simulink model "mRobotArm_PickAndPlace"  (R2021a)
settings: Solver=FixedStepAuto  StartTime=0.0  StopTime=inf  RelTol=1e-3  EnableMultiTasking=on
InitFcn:
  | initPoint=[pi/2 pi/2 pi/4 pi/4];
  | placePoint = [2.3562 1.1920 0.4461 0.0025];
  | pickPoint = [130; -130; 10];
undefined symbols (not defined in the file or in its folder): adHome6deg, adHome6rad, adWS
libraries: arduinolib x13, aerolibconvert2 x2
settings Model: SILPILModeSetting=veronly  ExtModeTrigDuration=2  Creator=loris  LastModifiedBy=angelo
settings OptimizationCC: EnhancedBackFolding=on  PassReuseOutputArgsAs=Individual arguments  ZeroExternalMemoryAtStartup=off  ZeroInternalMemoryAtStartup=off  MaxStackSize=64  OptimizeBlockOrder=speed  DifferentSizesBufferReuse=on  OptimizationCustomize=off  EfficientTunableParamExpr=on
settings DebuggingCC: ParameterTunabilityLossMsg=error
settings HardwareCC: ProdBitPerInt=16  ProdBitPerPointer=16  ProdBitPerSizeT=16  ProdBitPerPtrDiffT=16  ProdLargestAtomicFloat=None  ProdWordSize=8  ProdHWDeviceType=Atmel->AVR
settings SFSimCC: MATLABDynamicMemAlloc=off
settings RTWCC: SystemTargetFile=ert.tlc  HardwareBoard=Arduino Mega 2560  TemplateMakefile=ert_default_tmf  Toolchain=Arduino AVR  BuildConfiguration=Faster Runs
settings CodeAppCC: ForceParamTrailComments=on  IgnoreCustomStorageClasses=off  OperatorAnnotations=on  SimulinkDataObjDesc=on  SFDataObjDesc=on  InsertBlockDesc=on
settings ERTTargetCC: SupportContinuousTime=on  SupportVariableSizeSignals=on  ExtModeStaticAllocSize=2048

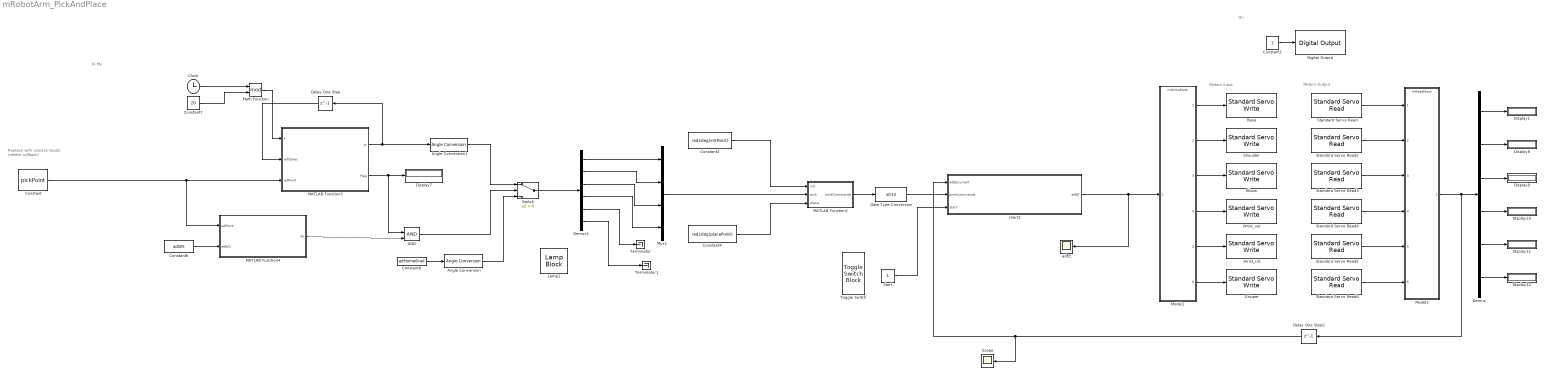
== system mRobotArm_PickAndPlace ==
  note: Replace with camera inputs
      | (delete callback)
  note: On
  note: Motors Output
  note: Motors Input
  note: IK My
  AND : Logic  IconShape=distinctive  AllPortsSameDT=off  OutDataTypeStr=boolean
  Angle Conversion : aerolibconvert2/Angle Conversion  IU=rad  OU=deg
  Angle Conversion1 : aerolibconvert2/Angle Conversion  IU=rad  OU=deg
  Base : arduinolib/Standard Servo Write  pinNumber=11  ServoIndex=0  blockPlatform=ARDUINO
  Clock : Clock
  Constant : Constant  Value=pickPoint
  Constant1 : Constant
  Constant3 : Constant  Value=rad2deg(initPoint)
  Constant4 : Constant  Value=rad2deg(placePoint)
  Constant6 : Constant  Value=adWS
  Constant7 : Constant  Value=20
  Constant8 : Constant  Value=adHome6rad
  Data Type Conversion : DataTypeConversion  OutDataTypeStr=int32
  Delay One Step : Delay  DelayLength=1  InitialCondition=adHome6rad  SampleTime=0.02
  Delay One Step2 : Delay  DelayLength=1  InitialCondition=adHome6deg
  Demux : Demux  Outputs=6
  Demux1 : Demux  Outputs=6
  Digital Output : arduinolib/Digital Output  pinNumber=12  Direction=output  blockPlatform=arduino
  Display{1,7..12} (7 alike) : Display
  Elbow : arduinolib/Standard Servo Write  pinNumber=9  ServoIndex=1  blockPlatform=ARDUINO
  Gripper : arduinolib/Standard Servo Write  pinNumber=3  ServoIndex=2  blockPlatform=ARDUINO
  Lamp1 : LampBlock  LabelPosition=Hide
  MATLAB Function1 : MATLAB Function  TreatAsAtomicUnit=on
  MATLAB Function3 : MATLAB Function  TreatAsAtomicUnit=on  SystemSampleTime=0.02
  MATLAB Function4 : MATLAB Function  TreatAsAtomicUnit=on  SystemSampleTime=0.02
  Math Function : Math  Operator=mod  SaturateOnIntegerOverflow=on
  Model1 : ModelReference  ModelNameDialog=mWriteMask.slx  SimulationMode=Normal  ModelReferenceVersion=1.1
  Model2 : ModelReference  ModelNameDialog=mReadMask.slx  SimulationMode=Normal  ModelReferenceVersion=1.1
  Mux1 : Mux
  Scope : Scope
  Shoulder : arduinolib/Standard Servo Write  pinNumber=10  ServoIndex=3  blockPlatform=ARDUINO
  Standard Servo Read : arduinolib/Standard Servo Read  pinNumber=11  SampleTime=0.02  ServoIndex=0  blockPlatform=ARDUINO
      settings: SourceProductBaseCode=ARDUINO
  Standard Servo Read2 : arduinolib/Standard Servo Read  pinNumber=10  SampleTime=0.02  ServoIndex=3  blockPlatform=ARDUINO
      settings: SourceProductBaseCode=ARDUINO
  Standard Servo Read3 : arduinolib/Standard Servo Read  pinNumber=9  SampleTime=0.02  ServoIndex=1  blockPlatform=ARDUINO
      settings: SourceProductBaseCode=ARDUINO
  Standard Servo Read4 : arduinolib/Standard Servo Read  pinNumber=6  SampleTime=0.02  ServoIndex=4  blockPlatform=ARDUINO
      settings: SourceProductBaseCode=ARDUINO
  Standard Servo Read5 : arduinolib/Standard Servo Read  pinNumber=5  SampleTime=0.02  ServoIndex=5  blockPlatform=ARDUINO
      settings: SourceProductBaseCode=ARDUINO
  Standard Servo Read6 : arduinolib/Standard Servo Read  pinNumber=3  SampleTime=0.02  ServoIndex=2  blockPlatform=ARDUINO
      settings: SourceProductBaseCode=ARDUINO
  Start : Constant
  Switch : Switch  Criteria=u2 > Threshold
  Terminator : Terminator
  Terminator1 : Terminator
  Toggle Switch : ToggleSwitchBlock  LabelPosition=Hide
      settings: Values={{'Off', 'On'}, [0 1]}
  Wrist_rot : arduinolib/Standard Servo Write  pinNumber=5  ServoIndex=5  blockPlatform=ARDUINO
  Wrist_ver : arduinolib/Standard Servo Write  pinNumber=6  ServoIndex=4  blockPlatform=ARDUINO
  adEE : Scope
  chart2 : Stateflow chart  TreatAsAtomicUnit=on  SystemSampleTime=0.02
  wires:
  Constant1/1 -> Digital Output/1
  Delay One Step2/1 -> Scope/1, chart2/1(adEEcurrent)
  Constant3/1 -> MATLAB Function1/1(init)
  Constant4/1 -> MATLAB Function1/3(place)
  MATLAB Function3/2(flag) -> Display7/1, AND/1
  Constant7/1 -> Math Function/2
  Constant6/1 -> MATLAB Function4/2(adWS)
  Clock/1 -> Math Function/1
  MATLAB Function3/1(jc) -> Delay One Step/1, Angle Conversion1/1
  Constant/1 -> MATLAB Function4/1(adPoint), MATLAB Function3/3(adPoint)
  Delay One Step/1 -> MATLAB Function3/2(adQprec)
  AND/1 -> Switch/2
  Math Function/1 -> MATLAB Function3/1(t)
  MATLAB Function4/1(ok) -> AND/2
  Demux1/1 -> Mux1/1
  Demux1/2 -> Mux1/2
  Demux1/3 -> Mux1/3
  Demux1/4 -> Mux1/4
  Mux1/1 -> MATLAB Function1/2(pick)
  Demux1/5 -> Terminator/1
  Switch/1 -> Demux1/1
  chart2/1(adEE) -> Model1/1, adEE/1
  Start/1 -> chart2/3(start)
  Demux/6 -> Display12/1
  Demux/2 -> Display8/1
  Demux/5 -> Display11/1
  Demux/4 -> Display10/1
  Demux/1 -> Display1/1
  Demux/3 -> Display9/1
  Model2/1 -> Delay One Step2/1, Demux/1
  Demux1/6 -> Terminator1/1
  MATLAB Function1/1(jointCommands) -> Data Type Conversion/1
  Data Type Conversion/1 -> chart2/2(JointCommands)
  Model1/1 -> Base/1
  Model1/2 -> Shoulder/1
  Model1/3 -> Elbow/1
  Model1/4 -> Wrist_ver/1
  Model1/5 -> Wrist_rot/1
  Model1/6 -> Gripper/1
  Standard Servo Read/1 -> Model2/1
  Standard Servo Read2/1 -> Model2/2
  Standard Servo Read3/1 -> Model2/3
  Standard Servo Read4/1 -> Model2/4
  Standard Servo Read5/1 -> Model2/5
  Standard Servo Read6/1 -> Model2/6
  Constant8/1 -> Angle Conversion/1
  Angle Conversion/1 -> Switch/3
  Angle Conversion1/1 -> Switch/1

== matlab function mRobotArm_PickAndPlace/MATLAB Function1 ==
  data: init input; pick input; jointCommands output; place input
function jointCommands = compose(init, pick, place)
jointCommands = [init'; pick'; init'; place'; init'];
end

== matlab function mRobotArm_PickAndPlace/MATLAB Function4 ==
  data: adPoint input; ok output; adWS input
function ok = verifierWS(adPoint, adWS)
ok = functions.isInsideWorkspace(adPoint, adWS(1), adWS(2), adWS(3));
end

== matlab function mRobotArm_PickAndPlace/MATLAB Function3 ==
  data: t input; adQprec input; adPoint input; jc output; flag output
function [jc, flag] = ikin(t, adQprec, adPoint)
if(t ~= 0)
    flag  	= true;
    jc      = adQprec;
    return;
end

% Joints definition
oJointBase      = classes.Joint(deg2rad(0)-pi/2, deg2rad(180)-pi/2);
oJointShoulder  = classes.Joint(deg2rad(15)-pi/2, deg2rad(165)-pi/2);
oJointElbow     = classes.Joint(deg2rad(0)-pi/2, deg2rad(180)-pi/2);
oJointPitch     = classes.Joint(deg2rad(0)-pi/2, deg2rad(180)-pi/2);
oJointWrist     = classes.Joint(deg2rad(0)-pi/2, deg2rad(180)-pi/2);

% Liks definition
% oLinkGround     = classes.Link(70);
% oLinkArm        = classes.Link(125);
% oLinkForearm    = classes.Link(125);
% oLinkHand       = classes.Link(185);

oLinkGround     = classes.Link(74);
oLinkArm        = classes.Link(125);
oLinkForearm    = classes.Link(125);
oLinkHand       = classes.Link(195);

% Braccio definition
oBraccio        = classes.Robot5Dof(oJointBase, oJointShoulder,     ...
                                    oJointElbow, oJointPitch,       ... 
                                    oJointWrist, oLinkGround,       ...
                                    oLinkArm, oLinkForearm,         ...
                                    oLinkHand);

% IKIN computation
[bOK, adQ]      = oBraccio.IKIN(adPoint);
% adQ(1)          = adQ(1)-pi/2; % FKIN non IKIN

% Output
jc              = [adQ+pi/2; 0; deg2rad(70)];
flag            = bOK;
end

== stateflow chart mRobotArm_PickAndPlace/chart2 ==
  settings: executeAtInitialization=1
  state WayPointReached
    entry:
    counter = 0;
    if currentState==2
    GripperDesired=50;
    grip = 1;
    elseif currentState==4
    GripperDesired=10;
    grip = 1;
    end
    during:
    % adEE=[adEE(1); adEE(2); adEE(3); adEE(4); adEE(5);nextStep(adEEcurrent(6),GripperDesired)];
    adEE(6) = nextStep(adEEcurrent(6),GripperDesired);
    counter = temporalCount(sec);
  state ToNextState
    entry:
    if currentState<5
    currentState=currentState+1;
    else
    stop=1;
    adEE = adEEcurrent;
    end
    grip = 0;
  state Init
    entry:
    grip = 0;
    currentState=1;
    stop=0;
    GripperDesired=10;
    du:adEE = adEEcurrent;
    %adEE = [90; 90; 45; 45; 0; 10];
  state ToNextPoint
    entry:
    adEEdesired=JointCommands(currentState,:)';
    during:
    adEE = [
    nextStep(adEEcurrent(1), adEEdesired(1));
    nextStep(adEEcurrent(2), adEEdesired(2));
    nextStep(adEEcurrent(3), adEEdesired(3));
    nextStep(adEEcurrent(4), adEEdesired(4));
    adEE(5);
    adEE(6)];
  (default) -> Init
  WayPointReached -> ToNextState : [ (grip==0) || ((grip==1) && (adEE(6) == GripperDesired) && (counter == 3)) ]
  Init -> ToNextPoint : [start == 1]
  ToNextState -> ToNextPoint : [stop==0]
  ToNextPoint -> WayPointReached : [all(adEEcurrent(1:4) == adEEdesired) ]
  data: current function_input; desired function_input; v function_output; current function_input; desired function_input; v function_output; adEEcurrent input; adEE output; adEEdesired local; currentState local; JointCommands input; stop local; start input; GripperDesired local; counter local; grip local
  function v = nextStep(current, desired):
    | function v = nextStep(current, desired)
    | if (current < desired)
    |     current = current + 1;
    | end
    | 
    | if (current > desired)
    |     current = current - 1;
    | end
    | 
    | v = current;
    | end
  function v = nextStep(current, desired):
    | function v = nextStep(current, desired)
    | if (current < desired)
    |     current = current + 1;
    | end
    | 
    | if (current > desired)
    |     current = current - 1;
    | end
    | 
    | v = current;
    | end
